simulink model "ego_stopped_lead_accelerating"  (R2025a)
settings: Solver=VariableStepAuto  StartTime=0.0  StopTime=10.0  RelTol=1e-3
settings Model: Creator=sanborkl  LastModifiedBy=sanborkl

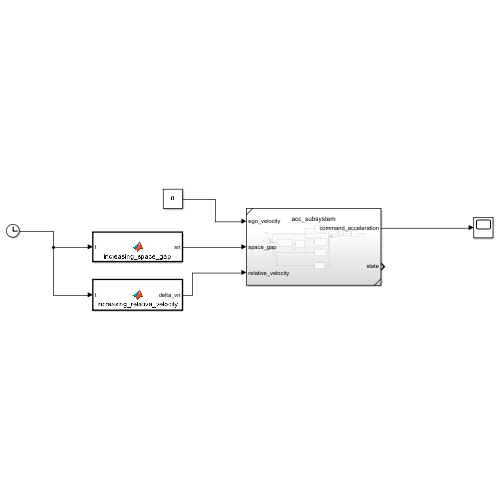
[thumbnail: Simulink's stored preview of the top-level diagram]
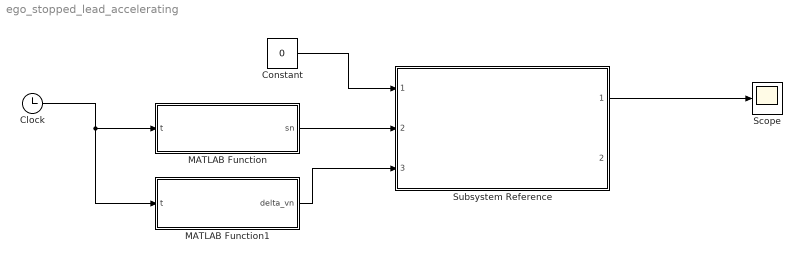
== system ego_stopped_lead_accelerating ==
  Clock : Clock
  Constant : Constant  Value=0
  MATLAB Function : MATLAB Function  TreatAsAtomicUnit=on
  MATLAB Function1 : MATLAB Function  TreatAsAtomicUnit=on
  Scope : Scope
      settings: ActiveDisplayYMinimum=0.5  ActiveDisplayYMaximum=2.5
  Subsystem Reference : Subsystem  ReferencedSubsystem=acc_subsystem
  wires:
  MATLAB Function1/1(delta_vn) -> Subsystem Reference/3
  MATLAB Function/1(sn) -> Subsystem Reference/2
  Subsystem Reference/1 -> Scope/1
  Constant/1 -> Subsystem Reference/1
  Clock/1 -> MATLAB Function1/1(t), MATLAB Function/1(t)

== matlab function ego_stopped_lead_accelerating/MATLAB Function1 ==
  data: t input; delta_vn output
function delta_vn = increasing_relative_velocity(t)

delta_vn = 2 * t;

== matlab function ego_stopped_lead_accelerating/MATLAB Function ==
  data: t input; sn output
function sn = increasing_space_gap(t)

sn = 3 * t + 20;
